simulink library "sm_rollerV_lib_contact_r9"  (R2023b)
settings: Solver=VariableStepAuto  StartTime=0.0  StopTime=10.0  RelTol=1e-3
undefined symbols (not defined in the file): L1, L2, L3, L4, L5, L6, L7, L8, L9, P1, P2, P3, P4, P5, P6, P7, P8, P9, S1, S2, Scene
libraries: sm_trackV_lib_terrain_contact x34, $bdroot x5
Description:
  | Copyright 2024 The MathWorks, Inc.
settings Model: Creator=smiller  LastModifiedBy=smiller

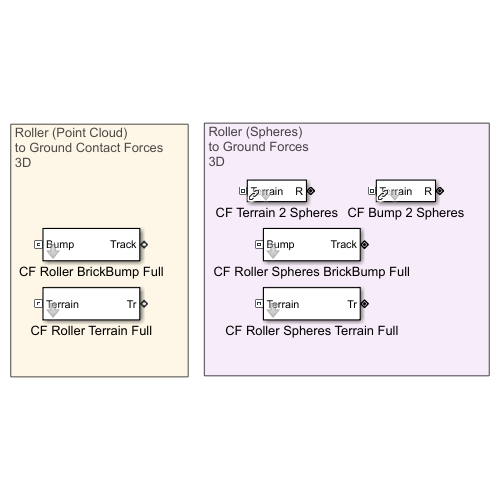
[thumbnail: Simulink's stored preview of the top-level diagram]
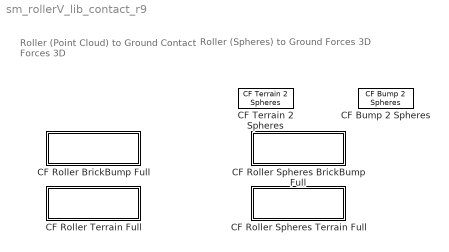
== system sm_rollerV_lib_contact_r9 ==
  note: Roller (Point Cloud)
      | to Ground Contact Forces
      | 3D
  note: Roller (Spheres)
      | to Ground Forces
      | 3D
  CF Bump 2 Spheres : sm_trackV_lib_terrain_contact/CF Bump 2 Spheres  K_BrickBump=Scene.Contact.BrickBump.K  B_BrickBump=Scene.Contact.BrickBump.B  TW_BrickBump=Scene.Contact.BrickBump.TW  CoefficientOfDynamicFriction=Scene.Contact.Terrain.mud  CoefficientOfStaticFriction=Scene.Contact.Terrain.mus  FrictionalCriticalVelocity=Scene.Contact.Terrain.CV
  CF Roller BrickBump Full : Subsystem  mask(Contact Forces, Rollers to Bump){K_BrickBump=Scene.Contact.BrickBump.K, B_BrickBump=Scene.Contact.BrickBump.B, TW_BrickBump=Scene.Contact.BrickBump.TW}
      mask prompts: K_BrickBump "Normal Stiffness (N/m)"; B_BrickBump "Normal Damping (N/(m/s))"; TW_BrickBump "Normal Transition Width (m)"
      mask help: Models contact force between rolling elements and bump.
  CF Roller Spheres BrickBump Full : Subsystem  mask(Contact Forces, Full Track to Bump){K_BrickBump=Scene.Contact.BrickBump.K, B_BrickBump=Scene.Contact.BrickBump.B, TW_BrickBump=Scene.Contact.BrickBump.TW}
      mask prompts: K_BrickBump "Normal Stiffness (N/m)"; B_BrickBump "Normal Damping (N/(m/s))"; TW_BrickBump "Normal Transition Width (m)"
      mask help: Models contact force between all spheres (two per rolling element) and a bump.
  CF Roller Spheres Terrain Full : Subsystem  mask(Contact Forces, All Rollers (Spheres) and Terrain)){K_Road=Scene.Contact.Terrain.K, B_Road=Scene.Contact.Terrain.B, TW_Road=Scene.Contact.Terrain.TW, F_dyn_Road=Scene.Contact.Terrain.mud, F_stat_Road=Scene.Contact.Terrain.mus, CV_Road=Scene.Contact.Terrain.CV}
      mask prompts: K_Road "Normal Stiffness (N/m)"; B_Road "Normal Damping (N/(m/s))"; TW_Road "Normal Transition Width (m)"; F_dyn_Road "Coefficient of Dynamic Friction"; F_stat_Road "Coefficient of Static Friction"; CV_Road "Critical Velocity (m/s)"
      mask help: Models contact force between all spheres (two per rolling element) and terrain.
  CF Roller Terrain Full : Subsystem  mask(Contact Forces, Rollers to Terrain){K_Road=Scene.Contact.Terrain.K, B_Road=Scene.Contact.Terrain.B, TW_Road=Scene.Contact.Terrain.TW, F_dyn_Road=Scene.Contact.Terrain.mud, F_stat_Road=Scene.Contact.Terrain.mus, CV_Road=Scene.Contact.Terrain.CV}
      mask prompts: K_Road "Normal Stiffness (N/m)"; B_Road "Normal Damping (N/(m/s))"; TW_Road "Normal Transition Width (m)"; F_dyn_Road "Coefficient of Dynamic Friction"; F_stat_Road "Coefficient of Static Friction"; CV_Road "Critical Velocity (m/s)"
      mask help: Models contact force between rolling elements and terrain.
  CF Terrain 2 Spheres : sm_trackV_lib_terrain_contact/CF Terrain 2 Spheres  NormalStiffness=Scene.Contact.Spheres.Terrain.K  NormalDamping=Scene.Contact.Spheres.Terrain.B  NormalTransitionRegionWidth=Scene.Contact.Spheres.Terrain.TW  CoefficientOfDynamicFriction=Scene.Contact.Spheres.Terrain.mud  CoefficientOfStaticFriction=Scene.Contact.Spheres.Terrain.mus  FrictionalCriticalVelocity=Scene.Contact.Spheres.Terrain.CV

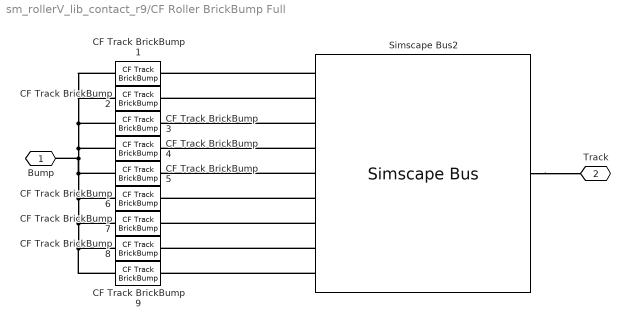
== system sm_rollerV_lib_contact_r9/CF Roller BrickBump Full ==
  CF Track BrickBump {1..9} (9 alike) : sm_trackV_lib_terrain_contact/CF Track BrickBump  NormalStiffness=K_BrickBump  NormalDamping=B_BrickBump  NormalTransitionRegionWidth=TW_BrickBump
      settings: LibrarySourceBlock=sm_chain_drive_lib/CF_BrickBump
  Simscape Bus2 : SimscapeBus  HierarchyStrings=P1;P2;P3;P4;P5;P6;P7;P8;P9  ConnectionType=Bus: CBO_Roller9
  Bump : PMIOPort  Side=Left
  Track : PMIOPort  Port=2  Side=Right
  connections:
  CF Track BrickBump 6/LConn1 -- CF Track BrickBump 7/LConn1 -- CF Track BrickBump 8/LConn1 -- CF Track BrickBump 9/LConn1 -- Bump/RConn1 -- CF Track BrickBump 1/LConn1 -- CF Track BrickBump 2/LConn1 -- CF Track BrickBump 3/LConn1 -- CF Track BrickBump 4/LConn1 -- CF Track BrickBump 5/LConn1
  Simscape Bus2/RConn1 -- Track/RConn1
  Simscape Bus2/LConn1 -- CF Track BrickBump 1/RConn1
  Simscape Bus2/LConn2 -- CF Track BrickBump 2/RConn1
  Simscape Bus2/LConn4 -- CF Track BrickBump 4/RConn1
  Simscape Bus2/LConn3 -- CF Track BrickBump 3/RConn1
  Simscape Bus2/LConn5 -- CF Track BrickBump 5/RConn1
  Simscape Bus2/LConn6 -- CF Track BrickBump 6/RConn1
  Simscape Bus2/LConn7 -- CF Track BrickBump 7/RConn1
  Simscape Bus2/LConn8 -- CF Track BrickBump 8/RConn1
  Simscape Bus2/LConn9 -- CF Track BrickBump 9/RConn1

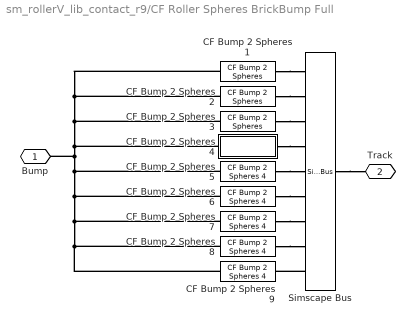
== system sm_rollerV_lib_contact_r9/CF Roller Spheres BrickBump Full ==
  CF Bump 2 Spheres 1 : sm_trackV_lib_terrain_contact/CF Bump 2 Spheres  K_BrickBump=K_BrickBump  B_BrickBump=B_BrickBump  TW_BrickBump=TW_BrickBump  CoefficientOfDynamicFriction=Scene.Contact.Terrain.mud  CoefficientOfStaticFriction=Scene.Contact.Terrain.mus  FrictionalCriticalVelocity=Scene.Contact.Terrain.CV
  CF Bump 2 Spheres 2 : sm_trackV_lib_terrain_contact/CF Bump 2 Spheres  K_BrickBump=K_BrickBump  B_BrickBump=B_BrickBump  TW_BrickBump=TW_BrickBump  CoefficientOfDynamicFriction=Scene.Contact.Terrain.mud  CoefficientOfStaticFriction=Scene.Contact.Terrain.mus  FrictionalCriticalVelocity=Scene.Contact.Terrain.CV
  CF Bump 2 Spheres 3 : sm_trackV_lib_terrain_contact/CF Bump 2 Spheres  K_BrickBump=K_BrickBump  B_BrickBump=B_BrickBump  TW_BrickBump=TW_BrickBump  CoefficientOfDynamicFriction=Scene.Contact.Terrain.mud  CoefficientOfStaticFriction=Scene.Contact.Terrain.mus  FrictionalCriticalVelocity=Scene.Contact.Terrain.CV
  CF Bump 2 Spheres 4 : Subsystem  mask{K_BrickBump=K_BrickBump, B_BrickBump=B_BrickBump, TW_BrickBump=TW_BrickBump}
      mask prompts: K_BrickBump "Normal Stiffness (N/m)"; B_BrickBump "Normal Damping (N/(m/s))"; TW_BrickBump "Normal Transition Width (m)"
      mask TypeOptions K_BrickBump: CF Bump Roller Sphere 1 /NormalStiffness | CF Bump Roller Sphere 2/NormalStiffness
      mask TypeOptions B_BrickBump: CF Bump Roller Sphere 1 /NormalDamping | CF Bump Roller Sphere 2/NormalDamping
      mask TypeOptions TW_BrickBump: CF Bump Roller Sphere 1 /NormalTransitionRegionWidth | CF Bump Roller Sphere 2/NormalTransitionRegionWidth
  CF Bump 2 Spheres {5..9} (5 alike) : $bdroot/CF Roller Spheres BrickBump Full/CF Bump 2 Spheres 4  K_BrickBump=K_BrickBump  B_BrickBump=B_BrickBump  TW_BrickBump=TW_BrickBump
  Simscape Bus : SimscapeBus  HierarchyStrings=L1;L2;L3;L4;L5;L6;L7;L8;L9
  Bump : PMIOPort  Side=Left
  Track : PMIOPort  Port=2  Side=Right
  connections:
  CF Bump 2 Spheres 1/RConn1 -- Simscape Bus/LConn1
  Simscape Bus/LConn9 -- CF Bump 2 Spheres 9/RConn1
  CF Bump 2 Spheres 5/RConn1 -- Simscape Bus/LConn5
  CF Bump 2 Spheres 3/RConn1 -- Simscape Bus/LConn3
  CF Bump 2 Spheres 6/RConn1 -- Simscape Bus/LConn6
  CF Bump 2 Spheres 7/RConn1 -- Simscape Bus/LConn7
  CF Bump 2 Spheres 8/RConn1 -- Simscape Bus/LConn8
  CF Bump 2 Spheres 2/RConn1 -- Simscape Bus/LConn2
  CF Bump 2 Spheres 4/RConn1 -- Simscape Bus/LConn4
  Simscape Bus/RConn1 -- Track/RConn1
  CF Bump 2 Spheres 9/LConn1 -- CF Bump 2 Spheres 8/LConn1 -- CF Bump 2 Spheres 7/LConn1 -- Bump/RConn1 -- CF Bump 2 Spheres 1/LConn1 -- CF Bump 2 Spheres 2/LConn1 -- CF Bump 2 Spheres 3/LConn1 -- CF Bump 2 Spheres 4/LConn1 -- CF Bump 2 Spheres 5/LConn1 -- CF Bump 2 Spheres 6/LConn1

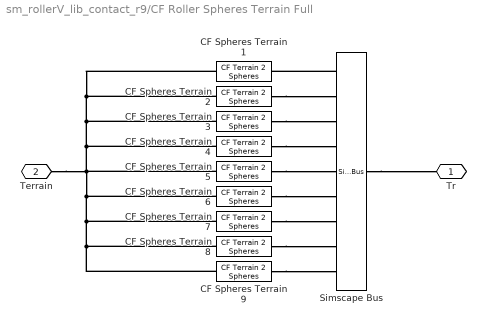
== system sm_rollerV_lib_contact_r9/CF Roller Spheres Terrain Full ==
  CF Spheres Terrain {1..9} (9 alike) : sm_trackV_lib_terrain_contact/CF Terrain 2 Spheres  NormalStiffness=K_Road  NormalDamping=B_Road  NormalTransitionRegionWidth=TW_Road  CoefficientOfDynamicFriction=F_dyn_Road  CoefficientOfStaticFriction=F_stat_Road  FrictionalCriticalVelocity=CV_Road
  Simscape Bus : SimscapeBus  HierarchyStrings=L1;L2;L3;L4;L5;L6;L7;L8;L9
  Tr : PMIOPort  Side=Right
  Terrain : PMIOPort  Port=2  Side=Left
  connections:
  CF Spheres Terrain 1/LConn1 -- CF Spheres Terrain 2/LConn1 -- CF Spheres Terrain 3/LConn1 -- CF Spheres Terrain 4/LConn1 -- Terrain/RConn1 -- CF Spheres Terrain 5/LConn1 -- CF Spheres Terrain 6/LConn1 -- CF Spheres Terrain 7/LConn1 -- CF Spheres Terrain 8/LConn1 -- CF Spheres Terrain 9/LConn1
  Simscape Bus/RConn1 -- Tr/RConn1
  Simscape Bus/LConn1 -- CF Spheres Terrain 1/RConn1
  CF Spheres Terrain 2/RConn1 -- Simscape Bus/LConn2
  CF Spheres Terrain 3/RConn1 -- Simscape Bus/LConn3
  CF Spheres Terrain 4/RConn1 -- Simscape Bus/LConn4
  CF Spheres Terrain 5/RConn1 -- Simscape Bus/LConn5
  CF Spheres Terrain 6/RConn1 -- Simscape Bus/LConn6
  CF Spheres Terrain 7/RConn1 -- Simscape Bus/LConn7
  CF Spheres Terrain 8/RConn1 -- Simscape Bus/LConn8
  CF Spheres Terrain 9/RConn1 -- Simscape Bus/LConn9

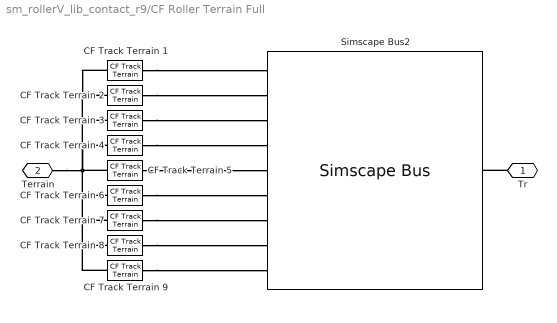
== system sm_rollerV_lib_contact_r9/CF Roller Terrain Full ==
  CF Track Terrain {1..9} (9 alike) : sm_trackV_lib_terrain_contact/CF Track Terrain  NormalStiffness=K_Road  NormalDamping=B_Road  NormalTransitionRegionWidth=TW_Road  CoefficientOfDynamicFriction=F_dyn_Road  CoefficientOfStaticFriction=F_stat_Road  FrictionalCriticalVelocity=CV_Road
      settings: LibrarySourceBlock=sm_chain_drive_lib/CF_Road
  Simscape Bus2 : SimscapeBus  HierarchyStrings=P1;P2;P3;P4;P5;P6;P7;P8;P9  ConnectionType=Bus: CBO_Roller9
  Tr : PMIOPort  Side=Right
  Terrain : PMIOPort  Port=2  Side=Left
  connections:
  CF Track Terrain 9/RConn1 -- Simscape Bus2/LConn9
  CF Track Terrain 1/LConn1 -- CF Track Terrain 2/LConn1 -- CF Track Terrain 3/LConn1 -- CF Track Terrain 4/LConn1 -- CF Track Terrain 5/LConn1 -- CF Track Terrain 6/LConn1 -- CF Track Terrain 7/LConn1 -- CF Track Terrain 9/LConn1 -- CF Track Terrain 8/LConn1 -- Terrain/RConn1
  CF Track Terrain 8/RConn1 -- Simscape Bus2/LConn8
  CF Track Terrain 3/RConn1 -- Simscape Bus2/LConn3
  CF Track Terrain 2/RConn1 -- Simscape Bus2/LConn2
  CF Track Terrain 1/RConn1 -- Simscape Bus2/LConn1
  CF Track Terrain 7/RConn1 -- Simscape Bus2/LConn7
  CF Track Terrain 5/RConn1 -- Simscape Bus2/LConn5
  CF Track Terrain 4/RConn1 -- Simscape Bus2/LConn4
  CF Track Terrain 6/RConn1 -- Simscape Bus2/LConn6
  Tr/RConn1 -- Simscape Bus2/RConn1

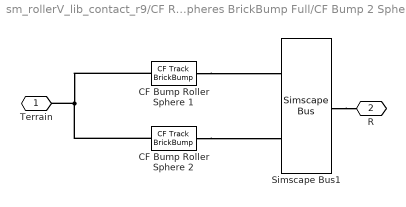
== system sm_rollerV_lib_contact_r9/CF Roller Spheres BrickBump Full/CF Bump 2 Spheres 4 ==
  "CF Bump Roller Sphere 1 " : sm_trackV_lib_terrain_contact/CF Track BrickBump  NormalStiffness=K_BrickBump  NormalDamping=B_BrickBump  NormalTransitionRegionWidth=TW_BrickBump
  CF Bump Roller Sphere 2 : sm_trackV_lib_terrain_contact/CF Track BrickBump  NormalStiffness=K_BrickBump  NormalDamping=B_BrickBump  NormalTransitionRegionWidth=TW_BrickBump
  Simscape Bus1 : SimscapeBus  HierarchyStrings=S1;S2
  Terrain : PMIOPort  Side=Left
  R : PMIOPort  Port=2  Side=Right
  connections:
  "CF Bump Roller Sphere 1 "/RConn1 -- Simscape Bus1/LConn1
  CF Bump Roller Sphere 2/LConn1 -- Terrain/RConn1 -- "CF Bump Roller Sphere 1 "/LConn1
  CF Bump Roller Sphere 2/RConn1 -- Simscape Bus1/LConn2
  Simscape Bus1/RConn1 -- R/RConn1
